simulink subsystem "s0507_alpha_theta_PP_polyfit"  (R2019b)
settings: Solver=VariableStepAuto  StartTime=0.0  StopTime=10.0  RelTol=1e-3
undefined symbols (not defined in the file): __PRM__SERIALIZED__DATA__, den_filter, dt_control, num_filter, PARAMS, SubsystemReferenceBlock
settings Model: Creator=francescoceresetti  LastModifiedBy=opc

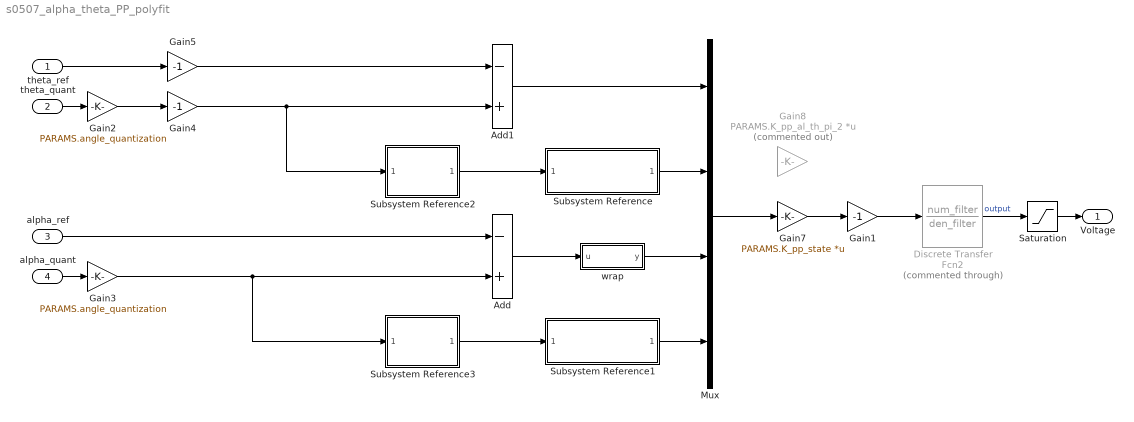
== system s0507_alpha_theta_PP_polyfit ==
  theta_ref : Inport
  theta_quant : Inport  Port=2
  alpha_ref : Inport  Port=3
  alpha_quant : Inport  Port=4
  Add : Sum  Inputs=-+
  Add1 : Sum  Inputs=-+
  Discrete Transfer Fcn2 : DiscreteTransferFcn  Commented=through  Numerator=num_filter  Denominator=den_filter  SampleTime=dt_control
  Gain1 : Gain  Gain=-1
  Gain2 : Gain  Gain=PARAMS.angle_quantization
  Gain3 : Gain  Gain=PARAMS.angle_quantization
  Gain4 : Gain  Gain=-1
  Gain5 : Gain  Gain=-1
  Gain7 : Gain  Gain=PARAMS.K_pp_state  Multiplication=Matrix(K*u)
  Gain8 : Gain  Commented=on  Gain=PARAMS.K_pp_al_th_pi_2  Multiplication=Matrix(K*u)
  Mux : Mux
  Saturation : Saturate  UpperLimit=PARAMS.V_sat  LowerLimit=-PARAMS.V_sat
  Subsystem Reference : Subsystem  BlockKeywords=__PRM__SERIALIZED__DATA__:SubsystemReferenceBlock  ReferencedSubsystem=Filtered_Derivative  num=num_der_filter  den=den_der_filter
  Subsystem Reference1 : Subsystem  BlockKeywords=__PRM__SERIALIZED__DATA__:SubsystemReferenceBlock  ReferencedSubsystem=Filtered_Derivative  num=num_der_filter  den=den_der_filter
  Subsystem Reference2 : Subsystem  BlockKeywords=__PRM__SERIALIZED__DATA__:SubsystemReferenceBlock  ReferencedSubsystem=Polynomial_Filter
  Subsystem Reference3 : Subsystem  BlockKeywords=__PRM__SERIALIZED__DATA__:SubsystemReferenceBlock  ReferencedSubsystem=Polynomial_Filter
  wrap : MATLAB Function  TreatAsAtomicUnit=on
  Voltage : Outport
  wires:
  alpha_quant/1 -> Gain3/1
  Mux/1 -> Gain7/1
  Gain7/1 -> Gain1/1
  Add1/1 -> Mux/1
  theta_quant/1 -> Gain2/1
  alpha_ref/1 -> Add/1
  Subsystem Reference1/1 -> Mux/4
  Subsystem Reference/1 -> Mux/2
  Add/1 -> wrap/1(u)
  wrap/1(y) -> Mux/3
  Saturation/1 -> Voltage/1
  Gain5/1 -> Add1/1
  theta_ref/1 -> Gain5/1
  Gain2/1 -> Gain4/1
  Discrete Transfer Fcn2/1 -> Saturation/1  "output"
  Gain1/1 -> Discrete Transfer Fcn2/1
  Gain4/1 -> Subsystem Reference2/1, Add1/2
  Gain3/1 -> Subsystem Reference3/1, Add/2
  Subsystem Reference2/1 -> Subsystem Reference/1
  Subsystem Reference3/1 -> Subsystem Reference1/1

== matlab function s0507_alpha_theta_PP_polyfit/wrap ==
  data: u input; y output
function y = wrap(u)
stop_condition = false;
y = u;
while ~stop_condition
    if y > pi
        y = y - 2*pi;
    elseif y < -pi
        y = y + 2*pi;
    else
        stop_condition = true;
    end
end
